simulink model "sldemo_auto_carelec"  (Simulink 10.0)
settings: Solver=ode23tb  StartTime=0.0  StopTime=3  MaxStep=0.001  RelTol=1e-4  EnableMultiTasking=on
libraries: powerlib x17
settings Model: Creator=The MathWorks Inc.  LastModifiedBy=bhisma  ExtModeTrigMode=oneshot  ExtModeArmWhenConnect=off
settings DataIOCC: SignalLoggingSaveFormat=ModelDataLogs  SignalLoggingName=sigsOut
settings OptimizationCC: BooleanDataType=off  ExpressionDepthLimit=2147483647  InitFltsAndDblsToZero=on  EfficientMapNaN2IntZero=off
settings DebuggingCC: SaveWithParameterizedLinksMsg=none  SignalResolutionControl=TryResolveAllWithWarning  MultiTaskDSMMsg=warning  MultiTaskCondExecSysMsg=none  FcnCallInpInsideContextMsg=warning  StateNameClashWarn=warning
settings GRTTargetCC: TargetFcnLib=ansi_tfl_tmw.mat  GeneratePreprocessorConditionals=Disable all
settings ConfigComp: CovExternalEMLEnable=off
settings SimscapeCC: SimscapeNormalizeSystem=off

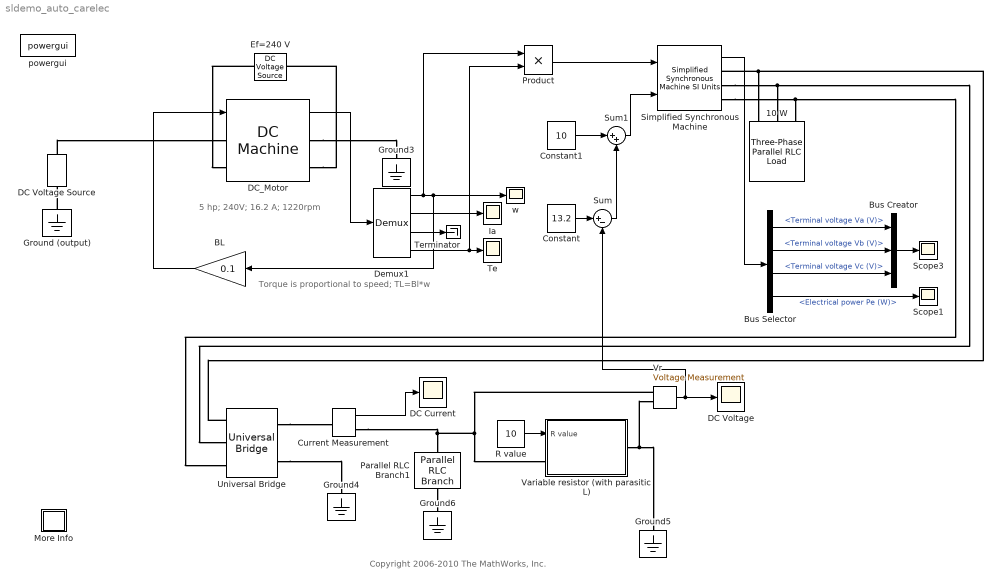
== system sldemo_auto_carelec ==
  note: 5 hp; 240V; 16.2 A; 1220rpm
  note: Torque is proportional to speed; TL=Bl*w
  note: Copyright 2006-2010 The MathWorks, Inc.
  10 W : powerlib/Elements/Three-Phase Parallel RLC Load  LConnTagsString=A|B|C  Configuration=Y (grounded)  NominalVoltage=20  Vabc=[1e3 1e3 1e3]  Vabcp=[1e3 1e3 1e3]  NominalFrequency=60  UnbalancedPower=off  ActivePower=1  InductivePower=0  CapacitivePower=0  Pabc=[10e3 9e3 11e3]  QLabc=[100 90 110]  QCabc=[100 90 110]  Pabcp=[10e3 9e3 11e3]  QLabcp=[100 90 110]  QCabcp=[100 90 110]  Measurements=None  LoadType=constant Z
      settings: SourceProductName=Simscape Electrical
  BL : Gain  Gain=0.1  SaturateOnIntegerOverflow=on  OutDataTypeStr=Inherit: Same as input  ParamDataTypeStr=Inherit: Same as input
  Bus Creator : BusCreator  Inputs=3
  Bus Selector : BusSelector  OutputSignals=Terminal voltage Va (V),Terminal voltage Vb (V),Terminal voltage Vc (V),Electrical power Pe (W)
  Constant : Constant  Value=13.2
  Constant1 : Constant  Value=10
  Current Measurement : powerlib/Measurements/Current Measurement  PhasorSimulation=off  OutputType=Magnitude  PSBequivalent=0
      settings: SourceProductName=Simscape Electrical
  DC Current : Scope
  DC Voltage : Scope
  DC Voltage Source : powerlib/Electrical Sources/DC Voltage Source  Amplitude=160  Measurements=None
      settings: SourceProductName=Simscape Electrical
  DC_Motor : powerlib/Machines/DC Machine  PresetModel=No  MechanicalLoad=Torque TL  FieldType=Wound  ShowDetailedParameters=on  MeasurementBus=off  RLa="[ 0.6  0.012]"  RLf="[ 240  120]"  Laf=1.8  MachineConstant=Torque constant (N.m/A)  Ke=1.8  Kt=1.8  J=1  Bm=0  Tf=0  w0=1  Ifinit=1  TsPowergui=0  TsBlock=-1
      settings: SourceProductName=Simscape Electrical
  Demux1 : Demux
  Ef=240 V : powerlib/Electrical Sources/DC Voltage Source  Amplitude=240  Measurements=None
      settings: SourceProductName=Simscape Electrical
  Ground (output) : powerlib/Elements/Ground  LConnTagsString=a
      settings: SourceProductName=Simscape Electrical
  Ground{3..6} (4 alike) : powerlib/Elements/Ground  LConnTagsString=a
      settings: SourceProductName=Simscape Electrical
  Ia : Scope
  More Info : Subsystem
      settings: OpenFcn=showdemo(bdroot(gcb))
      mask Display: disp('?')
  Parallel RLC Branch1 : powerlib/Elements/Parallel RLC Branch  LConnTagsString=a  RConnTagsString=__new0  BranchType=RC  Resistance=100  Inductance=1.0  SetiL0=off  InitialCurrent=0  Capacitance=50e-06  Setx0=off  InitialVoltage=0  Measurements=None
      settings: SourceProductName=Simscape Electrical
  Product : Product  SaturateOnIntegerOverflow=on  InputSameDT=on  OutDataTypeStr=Inherit: Same as first input
  R value : Constant  Value=10
  Scope1 : Scope
  Scope3 : Scope
  "Simplified Synchronous Machine " : powerlib/Machines/Simplified Synchronous Machine SI Units  ConnectionType=3-wire Y  MechanicalLoad=Mechanical power Pm  MeasurementBus=off  NominalParameters=[ 750, 20, 60 ]  Mechanical=[ inf, 0, 3]  InternalRL=[ 0.1, 2.15e-5 ]  InitialConditions="[ 0   0   0,0,0   0,0,0 ]"  IterativeDiscreteModel=Trapezoidal non iterative  TsBlock=-1  TsPowergui=0  LoadFlowParameters=[1,0,0,0,0]  Units=1  BusType=PV  Pref=0  Qref=0  Qmin=-inf  Qmax=+inf  PLF=0  QLF=0
      settings: SourceProductName=Simscape Electrical  SourceProductBaseCode=PS
  Sum : Sum  Inputs=|+-  SaturateOnIntegerOverflow=on  InputSameDT=on  OutDataTypeStr=Inherit: Same as first input
  Sum1 : Sum  Inputs=|++  SaturateOnIntegerOverflow=on  InputSameDT=on  OutDataTypeStr=Inherit: Same as first input
  Te : Scope
  Terminator : Terminator
  Universal Bridge : powerlib/Power Electronics/Universal Bridge  Arms=3  SnubberResistance=inf  SnubberCapacitance=100e-09  Device=Diodes  Ron=0.01  Lon=0  ForwardVoltages="[  0  0  ]"  ForwardVoltage=0.8  GTOparameters=[ 10e-6 , 20e-6 ]  IGBTparameters=[ 1e-6 , 2e-6 ]  Measurements=None  Measurements_2=None  converterType=Rectifier
      settings: SourceProductName=Simscape Electrical
  "Variable resistor (with parasitic L) " : Subsystem
      mask Display: disp('Variable Resistor');
  Vr : powerlib/Measurements/Voltage Measurement  PhasorSimulation=off  OutputType=Magnitude  PSBequivalent=0
      settings: SourceProductName=Simscape Electrical
  powergui : powerlib/powergui  SimulationMode=Continuous  SampleTime=0  frequency=60  Iterations=50  frequencyindice=0  Pbase=100e6  ErrMax=1e-4  UnitsV=kV  UnitsW=MW  buscounter=0  FunctionMessages=off  echomessages=off  EnableUseOfTLC=off  CurrentSourceSwitches=on  DisableSnubberDevices=off  DisableRonSwitches=off  DisableVfSwitches=off  DisplayEquations=off  AutomaticDiscreteSolvers=off  SolverType=Tustin  Interpol=off  ExternalGateDelay=off  methode=off  Ts=0  x0status=blocks  SPID=off  SwTol=0  HookPort=off  NonlinearTolerance=1e-4  nMaxIteration=100  ContinueOnMaxIteration=off  RestoreLinks=no  ResistiveCurrentMeasurement=off  Frange=[0:2:500]  Ylog=off  Xlog=on  ShowGrid=off  save=off  variable=ZData  structure=0  ZoomFFT=on  StartTime=0.0  cycles=1  DisplayStyle=1  fundamental=60  FreqAxis=off  MaxFrequency=1000  frequencyindicesteady=1  RmsSteady=1  display=off
      settings: SourceProductName=Simscape Electrical
  w : Scope
  wires:
  Demux1/3 -> Terminator/1
  Demux1/2 -> Ia/1
  Demux1/1 -> Product/1, BL/1, w/1
  Demux1/4 -> Te/1, Product/2
  Constant/1 -> Sum/1
  Constant1/1 -> Sum1/1
  Sum/1 -> Sum1/2
  R value/1 -> "Variable resistor (with parasitic L) "/1(R value)
  DC_Motor/1 -> Demux1/1
  BL/1 -> DC_Motor/1
  Product/1 -> "Simplified Synchronous Machine "/1
  "Simplified Synchronous Machine "/1 -> Bus Selector/1
  Bus Selector/4 -> Scope1/1  "<Electrical power Pe (W)>"
  Sum1/1 -> "Simplified Synchronous Machine "/2
  Vr/1 -> DC Voltage/1, Sum/2
  Current Measurement/1 -> DC Current/1
  Bus Selector/1 -> Bus Creator/1  "<Terminal voltage Va (V)>"
  Bus Selector/2 -> Bus Creator/2  "<Terminal voltage Vb (V)>"
  Bus Selector/3 -> Bus Creator/3  "<Terminal voltage Vc (V)>"
  Bus Creator/1 -> Scope3/1
  connections:
  DC_Motor/RConn1 -- Ground3/LConn1
  DC_Motor/RConn2 -- Ef=240 V/LConn1
  Ef=240 V/RConn1 -- DC_Motor/LConn2
  DC Voltage Source/RConn1 -- DC_Motor/LConn1
  Universal Bridge/RConn2 -- Ground4/LConn1
  Parallel RLC Branch1/RConn1 -- Ground6/LConn1
  Universal Bridge/RConn1 -- Current Measurement/LConn1
  Vr/LConn1 -- Current Measurement/RConn1 -- Parallel RLC Branch1/LConn1 -- "Variable resistor (with parasitic L) "/LConn1
  Ground (output)/LConn1 -- DC Voltage Source/LConn1
  "Variable resistor (with parasitic L) "/RConn1 -- Ground5/LConn1 -- Vr/LConn2
  Universal Bridge/LConn1 -- "Simplified Synchronous Machine "/RConn1 -- 10 W/LConn1
  "Simplified Synchronous Machine "/RConn2 -- Universal Bridge/LConn2 -- 10 W/LConn2
  "Simplified Synchronous Machine "/RConn3 -- Universal Bridge/LConn3 -- 10 W/LConn3

== system sldemo_auto_carelec/More Info ==

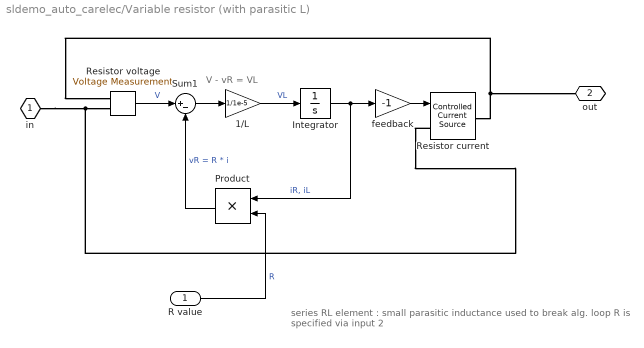
== system sldemo_auto_carelec/Variable resistor (with parasitic L)  ==
  note: V - vR = VL
  note: series RL element : small parasitic inductance used to break alg. loop
      | R is specified via input 2
  R value : Inport
  1/L : Gain  Gain=1/1e-5  SaturateOnIntegerOverflow=on  OutDataTypeStr=Inherit: Same as input  ParamDataTypeStr=Inherit: Same as input
  Integrator : Integrator  ZeroCross=off
  Product : Product  SaturateOnIntegerOverflow=on  InputSameDT=on  OutDataTypeStr=Inherit: Same as first input
  Resistor current : powerlib/Electrical Sources/Controlled Current Source  Initialize=on  Source_Type=AC  Amplitude=0  Phase=0  Frequency=0  Measurements=None
      settings: SourceProductName=Simscape Electrical
  Resistor voltage : powerlib/Measurements/Voltage Measurement  PhasorSimulation=off  OutputType=Magnitude  PSBequivalent=0
      settings: SourceProductName=Simscape Electrical
  Sum1 : Sum  Inputs=|+-  SaturateOnIntegerOverflow=on  InputSameDT=on  OutDataTypeStr=Inherit: Same as first input
  feedback : Gain  Gain=-1  SaturateOnIntegerOverflow=on  OutDataTypeStr=Inherit: Same as input  ParamDataTypeStr=Inherit: Same as input
  in : PMIOPort  Side=Left
  out : PMIOPort  Port=2  Side=Right
  wires:
  Sum1/1 -> 1/L/1
  Integrator/1 -> Product/1, feedback/1  "iR, iL"
  1/L/1 -> Integrator/1  "VL"
  R value/1 -> Product/2  "R"
  Product/1 -> Sum1/2  "vR = R * i"
  Resistor voltage/1 -> Sum1/1  "V"
  feedback/1 -> Resistor current/1
  connections:
  Resistor current/RConn1 -- out/RConn1 -- Resistor voltage/LConn1
  in/RConn1 -- Resistor voltage/LConn2 -- Resistor current/LConn1
